simulink model "task12"  (R2022b)
settings: Solver=FixedStepAuto  StartTime=0.0  StopTime=7  RelTol=1e-8
undefined symbols (not defined in the file): a0, a1, a2, k0, k1, y0, y1
settings Model: Creator=anton  LastModifiedBy=anton
settings DataIOCC: ExternalInput=data

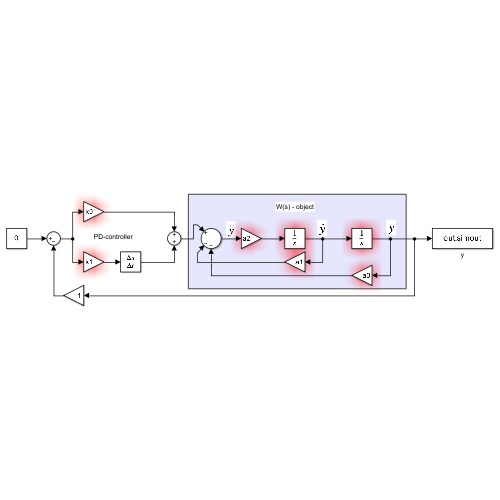
[thumbnail: Simulink's stored preview of the top-level diagram]
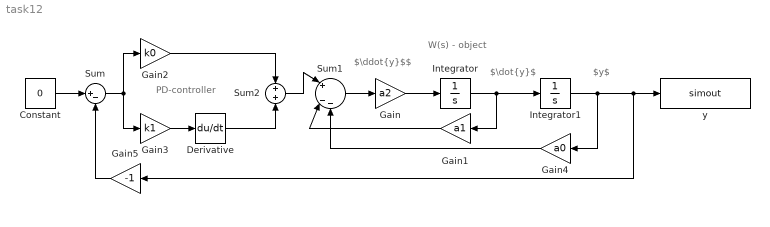
== system task12 ==
  note: $\ddot{y}$$
  note: W(s) - object
  note: PD-controller
  note: $\dot{y}$
  note: $y$
  Constant : Constant  Value=0
  Derivative : Derivative
  Gain : Gain  Gain=a2
  Gain1 : Gain  Gain=a1
  Gain2 : Gain  Gain=k0
  Gain3 : Gain  Gain=k1
  Gain4 : Gain  Gain=a0
  Gain5 : Gain  Gain=-1
  Integrator : Integrator  InitialCondition=y1
  Integrator1 : Integrator  InitialCondition=y0
  Sum : Sum  Inputs=|+-
  Sum1 : Sum  Inputs=|+|--
  Sum2 : Sum
  y : ToWorkspace  VariableName=simout  SaveFormat=Timeseries  SampleTime=-1
  wires:
  Constant/1 -> Sum/1
  Gain3/1 -> Derivative/1
  Gain2/1 -> Sum2/1
  Sum/1 -> Gain2/1, Gain3/1
  Integrator1/1 -> Gain4/1, y/1, Gain5/1
  Derivative/1 -> Sum2/2
  Sum2/1 -> Sum1/1
  Integrator/1 -> Gain1/1, Integrator1/1
  Sum1/1 -> Gain/1
  Gain/1 -> Integrator/1
  Gain1/1 -> Sum1/2
  Gain4/1 -> Sum1/3
  Gain5/1 -> Sum/2
